simulink model "BLDC_Hysteresis_Control"  (R2024b)
settings: Solver=VariableStepAuto  StartTime=0.0  StopTime=10  RelTol=1e-3
values from neighbouring files (symbols this model uses):
  iref = 70    [Parameters_List.m]
  pole_pair_number = 1    [Parameters_List.m]
  psim = 0.0175    [Parameters_List.m]
  Ts = 1e-4    (= 0.0001)    [Parameters_List.m]
  Tsc = 1e-4    (= 0.0001)    [Parameters_List.m]
  Vdc = 48    [Parameters_List.m]
libraries: fl_lib x15, nesl_utility x14, ee_lib x6, eeBldcCommutationLogic x1, eeHysteresisControl x1, eeGeneralControl x1
settings Model: Creator=subhajitroy005  LastModifiedBy=subhajitroy005

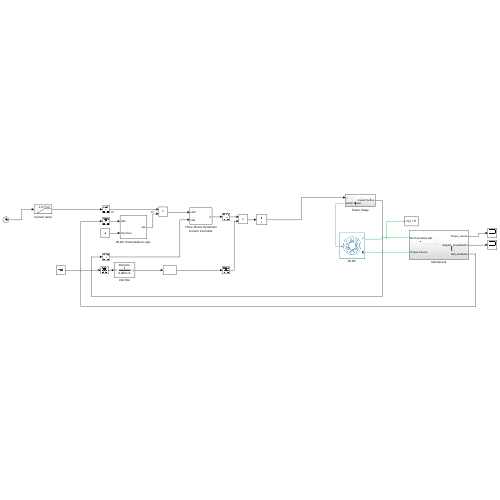
[thumbnail: Simulink's stored preview of the top-level diagram]
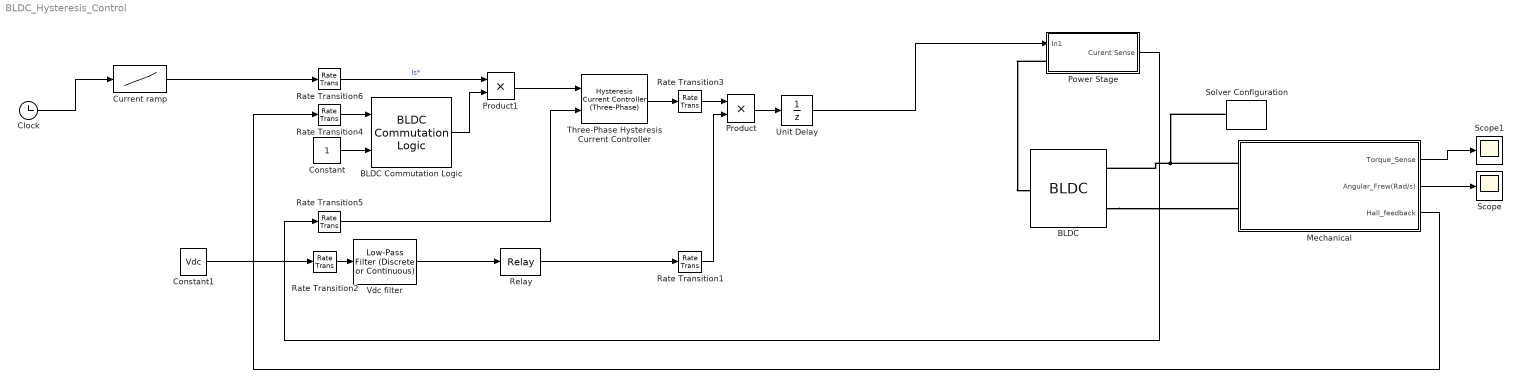
== system BLDC_Hysteresis_Control ==
  BLDC : ee_lib/Electromechanical/Permanent Magnet/BLDC  port_option=ee.enum.threePhasePort.composite  rotor_param=1  pm_flux_linkage=psim Wb  theta_constant=pi / (2*pole_pair_number) rad  emf_max=9.6 V  w_meas=600 rpm  DphiDtheta_tab=[0, -.1528, -.1528, .1528, .1528, 0] Wb/rad  back_emf_tab=[0, -9.6, -9.6, 9.6, 9.6, 0] V  rotor_angle_tab=[0, 7.5, 22.5, 37.5, 52.5, 60] deg  nPolePairs=pole_pair_number  axes_param=1  winding_type=ee.enum.statorconnection.wye  stator_param=2  machine_param=ee.enum.dqparameterization.constant  Ld=0.00022 H  Lq=0.00022 H  idVec=[-200, 0, 200] A  iqVec=[-200, 0, 200] A  LdMatrix=0.00022 * ones(3, 3) H  LqMatrix=0.00022 * ones(3, 3) H  L0=0.00016 H  Ls=Ls H  Lm=0 H  Ms=Ms H  Rs=Rs Ohm  zero_sequence=ee.enum.park.zerosequence.exclude  loss_param=ee.enum.ironloss.none  losses_oc=[0, 0, 0] W  losses_sc=[0, 0, 0] W  f_losses=60 Hz  Isc_losses=95 A  J=0 kg*m^2  lam=0 N*m/(rad/s)  i_d_specify=on  i_d_priority=High  i_d=0 A  i_d_nominal_specify=off  i_d_nominal_value=1  i_d_nominal_unit=A  i_q_specify=on  i_q_priority=High  i_q=0 A  i_q_nominal_specify=off  i_q_nominal_value=1  i_q_nominal_unit=A  torque_specify=off  torque_priority=None  torque=0 N*m  torque_nominal_specify=off  torque_nominal_value=1  torque_nominal_unit=N*m  angular_velocity_specify=off  angular_velocity_priority=High  angular_velocity=0 rpm  angular_velocity_nominal_specify=off  angular_velocity_nominal_value=1  angular_velocity_nominal_unit=rpm  angular_position_specify=off  angular_position_priority=High  angular_position=0 deg  angular_position_nominal_specify=off  angular_position_nominal_value=1  angular_position_nominal_unit=deg  alpha=3.93e-3 1/K  alpha_flux=-0.001 1/K  Tmeas=298.15 K  stator_thermal_mass=100 J/K  rotor_thermal_mass=200 J/K  Rm_percent_rotor=90  Rd_percent_rotor=30  temperatureA_specify=off  temperatureA_priority=High  temperatureA=25 degC  temperatureA_nominal_specify=off  temperatureA_nominal_value=1  temperatureA_nominal_unit=degC  temperatureB_specify=off  temperatureB_priority=High  temperatureB=25 degC  temperatureB_nominal_specify=off  temperatureB_nominal_value=1  temperatureB_nominal_unit=degC  temperatureC_specify=off  temperatureC_priority=High  temperatureC=25 degC  temperatureC_nominal_specify=off  temperatureC_nominal_value=1  temperatureC_nominal_unit=degC  temperatureR_specify=off  temperatureR_priority=High  temperatureR=25 degC  temperatureR_nominal_specify=off  temperatureR_nominal_value=1  temperatureR_nominal_unit=degC
      settings: InternalSimscapePortConfiguration="{\"Bottom\":[],\"Left\":[{\"id\":\"N\",\"label\":\"~\",\"type\":\"foundation.electrical.three_phase\"}],\"Right\":[{\"id\":\"R\",\"label\":\"R\",\"type\":\"foundation.mechanical.rotational.rotational\"},{\"id\":\"C\",\"label\":\"C\",\"type\":\"foundation.mechanical.rotational.rotational\"}],\"Top\":[]}"
  BLDC Commutation Logic : eeBldcCommutationLogic/BLDC Commutation Logic  Ts=Tsc
  Clock : Clock
  Constant : Constant
  Constant1 : Constant  Value=Vdc  VectorParams1D=off
  Current ramp : Lookup_n-D  NumberOfTableDimensions=1  BreakpointsForDimension1=[0 0.5 1]  Table=[0 iref iref]  InternalRulePriority=Speed  RndMeth=Simplest
  Mechanical : Subsystem
  Power Stage : Subsystem
  Product : Product
  Product1 : Product
  Rate Transition1 : RateTransition  OutPortSampleTime=Ts
  Rate Transition{2,4..6} (4 alike) : RateTransition  OutPortSampleTime=Tsc
  Rate Transition3 : RateTransition  OutPortSampleTime=Ts
  Relay : Relay  OnSwitchValue=Vdc/2  OffSwitchValue=Vdc/4
  Scope : Scope
  Scope1 : Scope
  Solver Configuration : nesl_utility/Solver Configuration  PhysicalDomain=network_engine_domain  SubClassName=solver  LeftPortType=input  RightPortType=generic  Tones=[]  Harmonics=[]  SimulateNoise=off  Profile=off  UseLocalSampling=off  EnableSwitchedLinearOptims=on  FrequencyDomain=off  UseCCode=off  RelTol=0.001  AbsTol=0.001  MinStep=1e-09  ToWorkspace=off  RevertToSquareIcSolve=off  NumHomotopyIterations=100  PhasorMode=off  PhasorModeNumHarmonics=1  ConsistencySolver=NEWTON_XTOL_AFTER_FTOL  IndexReductionMethod=DerivativeReplacement  DoDC=off  ResidualTolerance=1e-09  ConsistencyTolSource=GLOBAL  ConsistencyAbsTol=0.001  ConsistencyRelTol=0.001  ConsistencyTolFactor=1e-9  UseLocalSolver=on  LocalSolverChoice=NE_BACKWARD_EULER_ADVANCER  ResolveIndetEquations=on  FunctionEvalNumThread=1  LocalSolverSampleTime=Ts  DoFixedCost=on  MaxNonlinIter=5  MaxModeIter=2  ComputeImpulses=off  ImpulseIterations=2  LinearAlgebra=auto  LinearAlgebraNumThread=0  EquationFormulation=NE_TIME_EF  DelaysMemoryBudget=1024  AutomaticFiltering=on  FilteringTimeConstant=0.001  PartitionStorageMethod=AS_NEEDED  PartitionMemoryBudget=1024  PartitionMethod=ROBUST  MultibodyUseLocalSolver=off  MultibodyLocalSolverChoice=ODE1  MultibodyLocalSolverSampleTime=0.001
  Three-Phase Hysteresis Current Controller : eeHysteresisControl/Hysteresis Current Controller (Three-Phase)  h=h  Ts=Tsc
  Unit Delay : UnitDelay  SampleTime=Ts  HasFrameUpgradeWarning=on
  Vdc filter : eeGeneralControl/Low-Pass Filter (Discrete or Continuous)  K=1  T=0.005  B=inf  A=-inf  init_option=Inherited from block input  x0=0  Ts=Tsc
  wires:
  Clock/1 -> Current ramp/1
  BLDC Commutation Logic/1 -> Product1/2
  Rate Transition5/1 -> Three-Phase Hysteresis Current Controller/2
  Product1/1 -> Three-Phase Hysteresis Current Controller/1
  Rate Transition1/1 -> Product/2
  Relay/1 -> Rate Transition1/1
  Unit Delay/1 -> Power Stage/1(In1)
  Rate Transition4/1 -> BLDC Commutation Logic/1
  Constant/1 -> BLDC Commutation Logic/2
  Rate Transition6/1 -> Product1/1  "Is*"
  Three-Phase Hysteresis Current Controller/1 -> Rate Transition3/1
  Rate Transition2/1 -> Vdc filter/1
  Vdc filter/1 -> Relay/1
  Rate Transition3/1 -> Product/1
  Product/1 -> Unit Delay/1
  Mechanical/3(Hall_feedback) -> Rate Transition4/1
  Power Stage/1(Curent Sense) -> Rate Transition5/1
  Constant1/1 -> Rate Transition2/1
  Current ramp/1 -> Rate Transition6/1
  Mechanical/2(Angular_Frew(Rad/s)) -> Scope/1
  Mechanical/1(Torque_Sense) -> Scope1/1
  connections:
  Mechanical/LConn1 -- Solver Configuration/RConn1 -- BLDC/RConn2
  BLDC/RConn1 -- Mechanical/LConn2
  Power Stage/LConn1 -- BLDC/LConn1

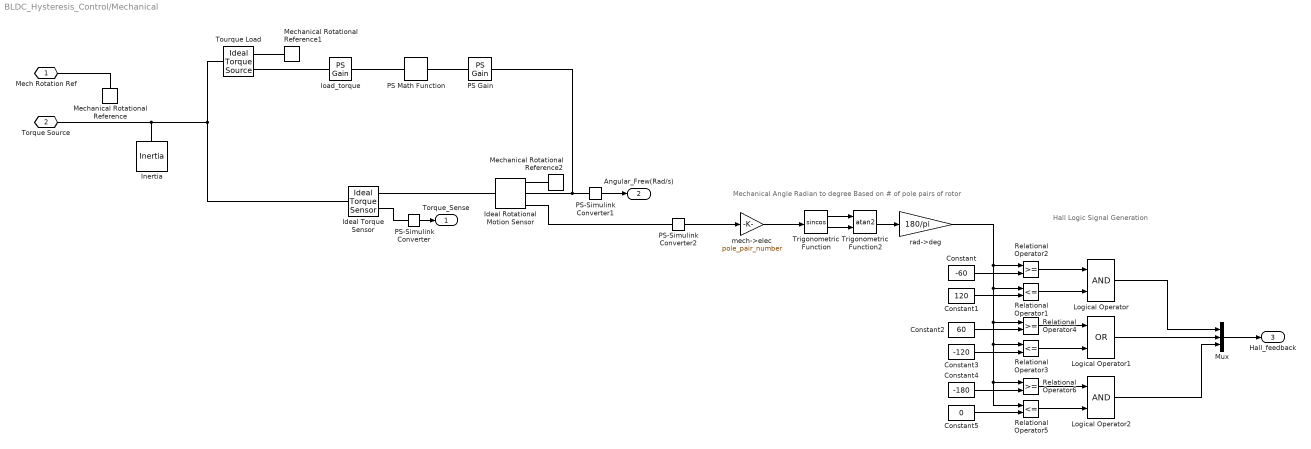
== system BLDC_Hysteresis_Control/Mechanical ==
  note: Hall Logic Signal Generation
  note: Mechanical Angle Radian to degree Based on # of pole pairs of rotor
  Constant : Constant  Value=-60
  Constant1 : Constant  Value=120
  Constant2 : Constant  Value=60
  Constant3 : Constant  Value=-120
  Constant4 : Constant  Value=-180
  Constant5 : Constant  Value=0
  Ideal Rotational Motion Sensor : fl_lib/Mechanical/Mechanical Sensors/Ideal Rotational Motion Sensor  reference=foundation.enum.MeasurementReference.difference  acceleration_port=false  velocity_port=true  position_port=true  wrap_angle=false  offset=0 rad
  Ideal Torque Sensor : fl_lib/Mechanical/Mechanical Sensors/Ideal Torque Sensor
  Inertia : fl_lib/Mechanical/Rotational Elements/Inertia  inertia=Jm kg*m^2  num_ports=foundation.enum.numPorts2.one  w_specify=on  w_priority=High  w=0 rad/s  w_nominal_specify=on  w_nominal_value=1  w_nominal_unit=rad/s  t_specify=off  t_priority=None  t=0 N*m  t_nominal_specify=off  t_nominal_value=1  t_nominal_unit=N*m
  Logical Operator : Logic  AllPortsSameDT=off  OutDataTypeStr=boolean
  Logical Operator1 : Logic  Operator=OR  AllPortsSameDT=off  OutDataTypeStr=boolean
  Logical Operator2 : Logic  AllPortsSameDT=off  OutDataTypeStr=boolean
  Mechanical Rotational Reference : fl_lib/Mechanical/Rotational Elements/Mechanical Rotational Reference
  Mechanical Rotational Reference1 : fl_lib/Mechanical/Rotational Elements/Mechanical Rotational Reference
  Mechanical Rotational Reference2 : fl_lib/Mechanical/Rotational Elements/Mechanical Rotational Reference
  Mux : Mux  Inputs=3
  PS Gain : fl_lib/Physical Signals/Functions/PS Gain  gain=1/200 1/(rad/s)
  PS Math Function : fl_lib/Physical Signals/Functions/PS Math Function  fcn_choice=7  v=1
  PS-Simulink Converter : nesl_utility/PS-Simulink Converter  PhysicalDomain=network_engine_domain  SubClassName=ps_output  LeftPortType=input  RightPortType=output  PseudoPeriodic=off  Frequencies=[]  VectorFormat=inherit  Unit=inherit  AffineConversion=off
  PS-Simulink Converter1 : nesl_utility/PS-Simulink Converter  PhysicalDomain=network_engine_domain  SubClassName=ps_output  LeftPortType=input  RightPortType=output  PseudoPeriodic=off  Frequencies=[]  VectorFormat=inherit  Unit=inherit  AffineConversion=off
  PS-Simulink Converter2 : nesl_utility/PS-Simulink Converter  PhysicalDomain=network_engine_domain  SubClassName=ps_output  LeftPortType=input  RightPortType=output  PseudoPeriodic=off  Frequencies=[]  VectorFormat=inherit  Unit=inherit  AffineConversion=off
  Relational Operator1 : RelationalOperator  Operator=<=
  Relational Operator2 : RelationalOperator
  Relational Operator3 : RelationalOperator  Operator=<=
  Relational Operator4 : RelationalOperator
  Relational Operator5 : RelationalOperator  Operator=<=
  Relational Operator6 : RelationalOperator
  Tourque Load : fl_lib/Mechanical/Mechanical Sources/Ideal Torque Source
  Trigonometric Function : Trigonometry  Operator=sincos
  Trigonometric Function2 : Trigonometry  Operator=atan2
  load_torque : fl_lib/Physical Signals/Functions/PS Gain  gain=-iref*psim*pole_pair_number*1.5 N*m
  mech->elec : Gain  Gain=pole_pair_number
  rad->deg : Gain  Gain=180/pi  SaturateOnIntegerOverflow=on  OutDataTypeStr=Inherit: Same as input  ParamDataTypeStr=Inherit: Same as input
  Mech Rotation Ref : PMIOPort  Side=Left
  Torque Source : PMIOPort  Port=2  Side=Left
  Torque_Sense : Outport
  Angular_Frew(Rad/s) : Outport  Port=2
  Hall_feedback : Outport  Port=3  VectorParamsAs1DForOutWhenUnconnected=off
  wires:
  PS-Simulink Converter/1 -> Torque_Sense/1
  PS-Simulink Converter1/1 -> Angular_Frew(Rad/s)/1
  Trigonometric Function2/1 -> rad->deg/1
  Trigonometric Function/1 -> Trigonometric Function2/1
  mech->elec/1 -> Trigonometric Function/1
  Trigonometric Function/2 -> Trigonometric Function2/2
  PS-Simulink Converter2/1 -> mech->elec/1
  Relational Operator5/1 -> Logical Operator2/2
  Constant2/1 -> Relational Operator4/2
  Relational Operator1/1 -> Logical Operator/2
  Logical Operator1/1 -> Mux/2
  Relational Operator3/1 -> Logical Operator1/2
  Logical Operator2/1 -> Mux/3
  Relational Operator6/1 -> Logical Operator2/1
  Constant1/1 -> Relational Operator1/2
  Constant4/1 -> Relational Operator6/2
  Constant3/1 -> Relational Operator3/2
  Logical Operator/1 -> Mux/1
  Constant/1 -> Relational Operator2/2
  Relational Operator4/1 -> Logical Operator1/1
  Relational Operator2/1 -> Logical Operator/1
  Constant5/1 -> Relational Operator5/2
  Mux/1 -> Hall_feedback/1
  rad->deg/1 -> Relational Operator4/1, Relational Operator3/1, Relational Operator5/1, Relational Operator6/1, Relational Operator1/1, Relational Operator2/1
  connections:
  Tourque Load/LConn1 -- Ideal Torque Sensor/LConn1 -- Torque Source/RConn1 -- Inertia/LConn1
  Mech Rotation Ref/RConn1 -- Mechanical Rotational Reference/LConn1
  Tourque Load/RConn2 -- Mechanical Rotational Reference1/LConn1
  Ideal Rotational Motion Sensor/LConn1 -- Ideal Torque Sensor/RConn1
  Ideal Torque Sensor/RConn2 -- PS-Simulink Converter/LConn1
  Ideal Rotational Motion Sensor/RConn2 -- PS Gain/LConn1 -- PS-Simulink Converter1/LConn1
  Mechanical Rotational Reference2/LConn1 -- Ideal Rotational Motion Sensor/RConn1
  PS-Simulink Converter2/LConn1 -- Ideal Rotational Motion Sensor/RConn3
  PS Gain/RConn1 -- PS Math Function/LConn1
  load_torque/LConn1 -- PS Math Function/RConn1
  Tourque Load/RConn1 -- load_torque/RConn1

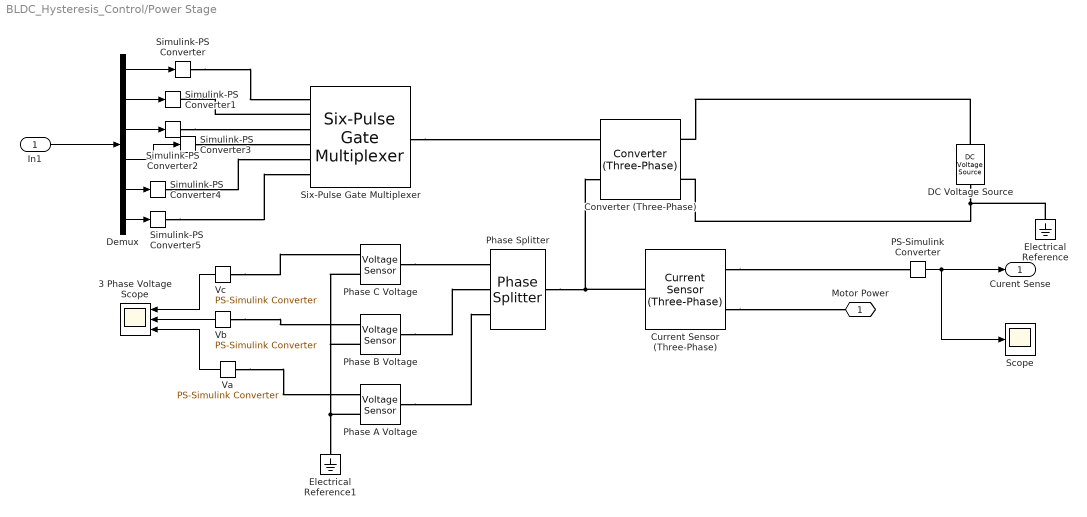
== system BLDC_Hysteresis_Control/Power Stage ==
  In1 : Inport
  3 Phase Voltage Scope : Scope  NumInputPorts=3
  Converter (Three-Phase) : ee_lib/Semiconductors & Converters/Converters/Converter (Three-Phase)  port_option=ee.enum.threePhasePort.composite  fidelity_option=ee.enum.converters.fidelity.detailed  device_type=ee.enum.converters.switchingdevice.igbt  showThermalPort=false  K=0  Vth=0.5 V  Vgt=1 V  Vgt_off=-1 V  Ih=1 A  Vf=0.8 V  Ron=0.001 Ohm  Rds=0.001 Ohm  Goff=1e-5 1/Ohm  Eon_scalar=22.86e-3 J  Eoff_scalar=17.14e-3 J  Eoff_natural_commutation=10e-3 J  Voff=300 V  Iout_scalar=600 A  onCurrentMeasDelay=0 s  useCurrentFromPreviousCycle=false  useVoltageFromPreviousCycle=false  diode_param=ee.enum.converters.protectiondiode.nodynamics  diode_Vf=0.8 V  diode_Ron=0.001 Ohm  diode_Goff=1e-5 1/Ohm  diode_C=50 nF  diode_iRM=-235 A  diode_iF=300 A  diode_idot=-50 A/us  diode_trr_param=ee.enum.converters.diodetrr.trr_factor  diode_trr_factor=3  diode_trr=15 us  diode_Qrr=1500 s*uA  diode_rec_loss_model=ee.enum.diode.reverseRecoveryModel.fixed  diode_ErecVal=0 J  diode_scaleWithIandV=false  diode_ErecMat=zeros(2, 3) J  diode_TjrecVec=[298.15, 398.15] K  diode_IfrecVec=[.1, 1, 10] A  diode_IrecVal=10 A  diode_VrecVal=10 V  diode_tFilter=1 / 1000 / 100 s  thermal_network_parameterization=ee.enum.thermalNetworkTopology.external  Rth=[.08, .5] K/W  Rth_Cauer=[.08, .1, .5] K/W  Rth_Foster=[.08, .14, .22, .16] K/W  thermal_mass_parameterization=ee.enum.thermalNetwork.timeconstant  thermal_mass=[.01, .5] J/K  thermal_mass_Cauer=[.01, .1, .5] J/K  thermal_mass_Foster=[.001, .005, .05, .5] J/K  thermal_time_constant=[.001, .2] s  thermal_time_constant_Cauer=[.001, .1, .2] s  thermal_time_constant_Foster=[7e-05, .0007, .01, .08] s  thermal_mass_initial_temperatures=[25, 25] degC  thermal_mass_initial_temperatures_Cauer=[25, 25, 25] degC  junction_thermal_mass=0.01 J/K  Tvec_initial_Foster=[25, 25, 25, 25] degC  snubber_type=ee.enum.converters.snubber.exclude  Cs=1e-7 F  Rs=0.1 Ohm  Vce_loss=[0, 150, 300] V
  Current Sensor (Three-Phase) : ee_lib/Sensors & Transducers/Current Sensor (Three-Phase)
  DC Voltage Source : ee_lib/Additional Components/SPICE Sources/DC Voltage Source  DC=Vdc V
  Demux : Demux  Outputs=6
  Electrical Reference : fl_lib/Electrical/Electrical Elements/Electrical Reference
  Electrical Reference1 : fl_lib/Electrical/Electrical Elements/Electrical Reference
  PS-Simulink Converter : nesl_utility/PS-Simulink Converter  PhysicalDomain=network_engine_domain  SubClassName=ps_output  LeftPortType=input  RightPortType=output  PseudoPeriodic=off  Frequencies=[]  VectorFormat=inherit  Unit=inherit  AffineConversion=off
  Phase A Voltage : fl_lib/Electrical/Electrical Sensors/Voltage Sensor
  Phase B Voltage : fl_lib/Electrical/Electrical Sensors/Voltage Sensor
  Phase C Voltage : fl_lib/Electrical/Electrical Sensors/Voltage Sensor
  Phase Splitter : ee_lib/Connectors & References/Phase Splitter
  Scope : Scope
  Simulink-PS Converter{,1..5} (6 alike) : nesl_utility/Simulink-PS Converter  PhysicalDomain=network_engine_domain  SubClassName=ps_input  LeftPortType=input  RightPortType=output  PseudoPeriodic=off  Frequencies=[]  NoiseDistribution=none  NoiseParameters=[]  Unit=1  AffineConversion=off  FilteringAndDerivatives=provide  SimscapeFilterOrder=1  InputFilterTimeConstant=0.001  UdotUserProvided=0
  Six-Pulse Gate Multiplexer : ee_lib/Semiconductors & Converters/Converters/Six-Pulse Gate Multiplexer  port_option=ee.enum.controlport.ps
  Va : nesl_utility/PS-Simulink Converter  PhysicalDomain=network_engine_domain  SubClassName=ps_output  LeftPortType=input  RightPortType=output  PseudoPeriodic=off  Frequencies=[]  VectorFormat=inherit  Unit=inherit  AffineConversion=off
  Vb : nesl_utility/PS-Simulink Converter  PhysicalDomain=network_engine_domain  SubClassName=ps_output  LeftPortType=input  RightPortType=output  PseudoPeriodic=off  Frequencies=[]  VectorFormat=inherit  Unit=inherit  AffineConversion=off
  Vc : nesl_utility/PS-Simulink Converter  PhysicalDomain=network_engine_domain  SubClassName=ps_output  LeftPortType=input  RightPortType=output  PseudoPeriodic=off  Frequencies=[]  VectorFormat=inherit  Unit=inherit  AffineConversion=off
  Motor Power : PMIOPort  Side=Left
  Curent Sense : Outport
  wires:
  Demux/1 -> Simulink-PS Converter/1
  Demux/3 -> Simulink-PS Converter2/1
  Demux/2 -> Simulink-PS Converter1/1
  Demux/4 -> Simulink-PS Converter3/1
  Demux/5 -> Simulink-PS Converter4/1
  Demux/6 -> Simulink-PS Converter5/1
  Vc/1 -> 3 Phase Voltage Scope/1
  Vb/1 -> 3 Phase Voltage Scope/2
  Va/1 -> 3 Phase Voltage Scope/3
  PS-Simulink Converter/1 -> Scope/1, Curent Sense/1
  In1/1 -> Demux/1
  connections:
  DC Voltage Source/LConn1 -- Converter (Three-Phase)/RConn1
  DC Voltage Source/RConn1 -- Electrical Reference/LConn1 -- Converter (Three-Phase)/RConn2
  Six-Pulse Gate Multiplexer/RConn1 -- Converter (Three-Phase)/LConn1
  Simulink-PS Converter/RConn1 -- Six-Pulse Gate Multiplexer/LConn1
  Simulink-PS Converter2/RConn1 -- Six-Pulse Gate Multiplexer/LConn3
  Six-Pulse Gate Multiplexer/LConn2 -- Simulink-PS Converter1/RConn1
  Simulink-PS Converter3/RConn1 -- Six-Pulse Gate Multiplexer/LConn4
  Simulink-PS Converter4/RConn1 -- Six-Pulse Gate Multiplexer/LConn5
  Simulink-PS Converter5/RConn1 -- Six-Pulse Gate Multiplexer/LConn6
  Phase Splitter/LConn1 -- Current Sensor (Three-Phase)/LConn1 -- Converter (Three-Phase)/LConn2
  Phase C Voltage/LConn1 -- Phase Splitter/RConn3
  Phase B Voltage/LConn1 -- Phase Splitter/RConn2
  Phase A Voltage/LConn1 -- Phase Splitter/RConn1
  Phase A Voltage/RConn2 -- Phase C Voltage/RConn2 -- Phase B Voltage/RConn2 -- Electrical Reference1/LConn1
  Vc/LConn1 -- Phase C Voltage/RConn1
  Vb/LConn1 -- Phase B Voltage/RConn1
  Va/LConn1 -- Phase A Voltage/RConn1
  Current Sensor (Three-Phase)/RConn2 -- Motor Power/RConn1
  Current Sensor (Three-Phase)/RConn1 -- PS-Simulink Converter/LConn1
